simulink model "PIDDynamics (2)"  (R2017a)
settings: Solver=ode113  StartTime=0.0  StopTime=1.3  RelTol=1e-3
settings Model: Creator=dvelas25  LastModifiedBy=dvelas25

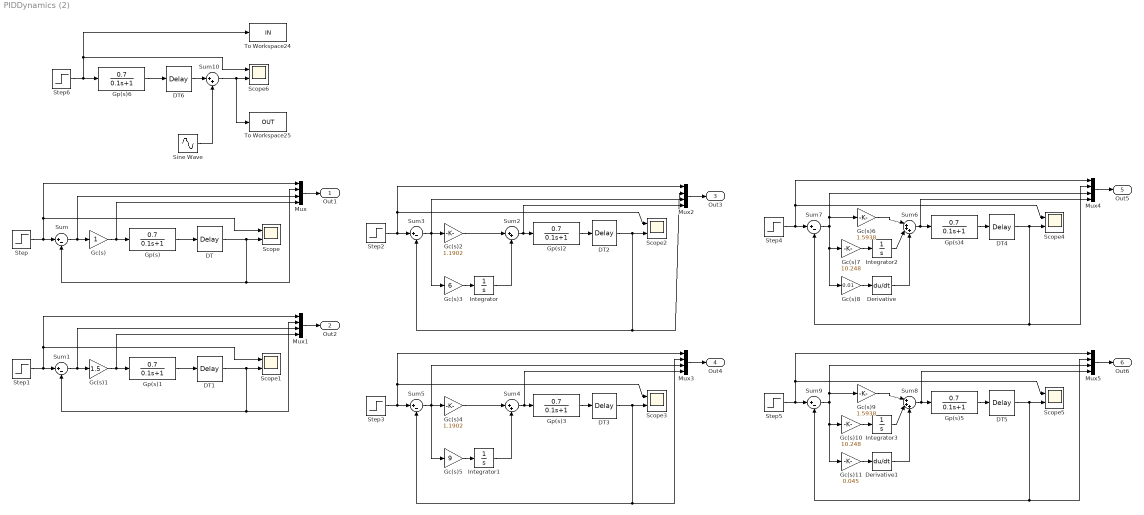
== system PIDDynamics (2) ==
  DT{,1..6} (7 alike) : TransportDelay  DelayTime=0.1
  Derivative : Derivative
  Derivative1 : Derivative
  Gc(s) : Gain
  Gc(s)1 : Gain  Gain=1.5
  Gc(s)10 : Gain  Gain=10.248
  Gc(s)11 : Gain  Gain=0.045
  Gc(s)2 : Gain  Gain=1.1902
  Gc(s)3 : Gain  Gain=6
  Gc(s)4 : Gain  Gain=1.1902
  Gc(s)5 : Gain  Gain=9
  Gc(s)6 : Gain  Gain=1.5938
  Gc(s)7 : Gain  Gain=10.248
  Gc(s)8 : Gain  Gain=0.01
  Gc(s)9 : Gain  Gain=1.5938
  Gp(s){,1..6} (7 alike) : TransferFcn  Numerator=[0.7]  Denominator=[0.1 1]
  Integrator{,1..3} (4 alike) : Integrator
  Mux{,1..5} (6 alike) : Mux
  Scope{,1..6} (7 alike) : Scope  NumInputPorts=2
  Sine Wave : Sin  Amplitude=0.005  Frequency=500  SampleTime=0
  Step{,1..6} (7 alike) : Step  Time=0.1  SampleTime=0
  Sum{,1,3,5,7,9} (6 alike) : Sum  Inputs=|+-
  Sum10 : Sum  Inputs=|++
  Sum2 : Sum  Inputs=|++
  Sum4 : Sum  Inputs=|++
  Sum6 : Sum  Inputs=|+++
  Sum8 : Sum  Inputs=|+++
  To Workspace24 : ToWorkspace  VariableName=IN  SaveFormat=Timeseries  SampleTime=-1
  To Workspace25 : ToWorkspace  VariableName=OUT  SaveFormat=Timeseries  SampleTime=-1
  Out1 : Outport  SignalName=SYSA1
  Out2 : Outport  Port=2  SignalName=SYSA2
  Out3 : Outport  Port=3  SignalName=SYSB1
  Out4 : Outport  Port=4  SignalName=SYSB2
  Out5 : Outport  Port=5  SignalName=SYSC1
  Out6 : Outport  Port=6  SignalName=SYSC2
  wires:
  DT/1 -> Scope/2, Mux/2, Sum/2
  Gp(s)/1 -> DT/1
  Step/1 -> Mux/1, Scope/1, Sum/1
  Sum/1 -> Mux/3, Gc(s)/1
  Gc(s)/1 -> Mux/4, Gp(s)/1
  Gc(s)1/1 -> Mux1/4, Gp(s)1/1
  Sum1/1 -> Mux1/3, Gc(s)1/1
  Step1/1 -> Sum1/1, Mux1/1, Scope1/1
  Gp(s)1/1 -> DT1/1
  DT1/1 -> Sum1/2, Mux1/2, Scope1/2
  DT2/1 -> Sum3/2, Mux2/2, Scope2/2
  Step2/1 -> Sum3/1, Mux2/1, Scope2/1
  Sum3/1 -> Mux2/3, Gc(s)3/1, Gc(s)2/1
  Gp(s)2/1 -> DT2/1
  Gc(s)3/1 -> Integrator/1
  Gc(s)2/1 -> Sum2/1
  Sum2/1 -> Mux2/4, Gp(s)2/1
  Integrator/1 -> Sum2/2
  Integrator1/1 -> Sum4/2
  Sum4/1 -> Mux3/4, Gp(s)3/1
  Gc(s)4/1 -> Sum4/1
  Gc(s)5/1 -> Integrator1/1
  Gp(s)3/1 -> DT3/1
  Sum5/1 -> Mux3/3, Gc(s)4/1, Gc(s)5/1
  Step3/1 -> Mux3/1, Scope3/1, Sum5/1
  Integrator2/1 -> Sum6/2
  Sum6/1 -> Mux4/4, Gp(s)4/1
  Gc(s)6/1 -> Sum6/1
  Gc(s)7/1 -> Integrator2/1
  Gp(s)4/1 -> DT4/1
  Sum7/1 -> Mux4/3, Gc(s)6/1, Gc(s)8/1, Gc(s)7/1
  Step4/1 -> Mux4/1, Scope4/1, Sum7/1
  Gc(s)8/1 -> Derivative/1
  Derivative/1 -> Sum6/3
  Derivative1/1 -> Sum8/3
  Gc(s)11/1 -> Derivative1/1
  DT5/1 -> Scope5/2, Mux5/2, Sum9/2
  Step5/1 -> Sum9/1, Mux5/1, Scope5/1
  Sum9/1 -> Gc(s)10/1, Gc(s)11/1, Gc(s)9/1, Mux5/3
  Gp(s)5/1 -> DT5/1
  Gc(s)10/1 -> Integrator3/1
  Gc(s)9/1 -> Sum8/1
  Sum8/1 -> Mux5/4, Gp(s)5/1
  Integrator3/1 -> Sum8/2
  Step6/1 -> Gp(s)6/1, To Workspace24/1, Scope6/1
  Gp(s)6/1 -> DT6/1
  DT6/1 -> Sum10/1
  Sine Wave/1 -> Sum10/2
  Sum10/1 -> To Workspace25/1, Scope6/2
  Mux/1 -> Out1/1
  Mux1/1 -> Out2/1
  Mux2/1 -> Out3/1
  Mux3/1 -> Out4/1
  Mux4/1 -> Out5/1
  Mux5/1 -> Out6/1
  DT3/1 -> Sum5/2, Mux3/2, Scope3/2
  DT4/1 -> Sum7/2, Mux4/2, Scope4/2
